simulink model "LoadFlow116BusNetwork_original"  (R2024a)
settings: Solver=FixedStepDiscrete  StartTime=0.0  StopTime=4.5  FixedStep=75e-6  RelTol=1e-3  EnableMultiTasking=on
undefined symbols (not defined in the file or in its folder): D1, D11, Delta
libraries: spsSeriesRLCBranchLib x164, spsLoadFlowBusLib x116, spsDistributedParametersLineLib x79, spsThreePhaseSeriesRLCLoadLib x60, spsThreePhaseTransformerTwoWindingsLib x52, spsThreePhaseParallelRLCLoadLib x44, spsThreePhaseVIMeasurementLib x44, spsSynchronousMachinepuStandardLib x28, spsExcitationSystemLib x28, spsHydraulicTurbineandGovernorLib x28, spsGenericPowerSystemStabilizerLib x28, spsMultiBandPowerSystemStabilizerLib x28
(part 7 of 15)

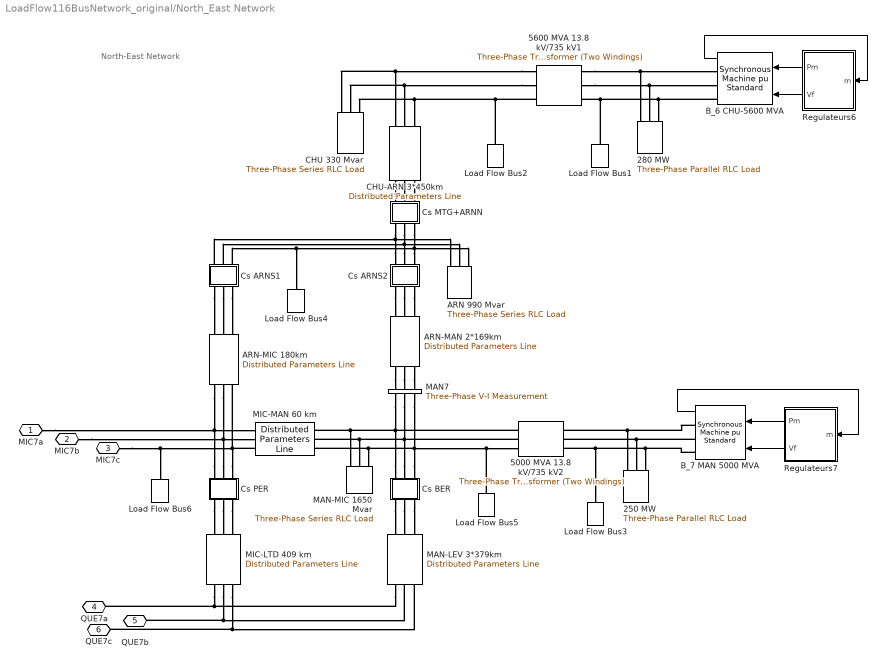
== system LoadFlow116BusNetwork_original/North_East Network ==
  note: North-East Network
  250 MW : spsThreePhaseParallelRLCLoadLib/Three-Phase Parallel RLC Load  LConnTagsString=A|B|C  Configuration=Y (grounded)  NominalVoltage=(13800)*1  Vabc=[1e3 1e3 1e3]  Vabcp=[1e3 1e3 1e3]  NominalFrequency=60  UnbalancedPower=off  ActivePower=250000000  InductivePower=0  CapacitivePower=0  Pabc=[10e3 9e3 11e3]  QLabc=[100 90 110]  QCabc=[100 90 110]  Pabcp=[10e3 9e3 11e3]  QLabcp=[100 90 110]  QCabcp=[100 90 110]  Measurements=None  LoadType=constant PQ
  280 MW : spsThreePhaseParallelRLCLoadLib/Three-Phase Parallel RLC Load  LConnTagsString=A|B|C  Configuration=Y (grounded)  NominalVoltage=(13800)*1  Vabc=[1e3 1e3 1e3]  Vabcp=[1e3 1e3 1e3]  NominalFrequency=60  UnbalancedPower=off  ActivePower=280000000  InductivePower=0  CapacitivePower=0  Pabc=[10e3 9e3 11e3]  QLabc=[100 90 110]  QCabc=[100 90 110]  Pabcp=[10e3 9e3 11e3]  QLabcp=[100 90 110]  QCabcp=[100 90 110]  Measurements=None  LoadType=constant PQ
  5000 MVA 13.8 kV/735 kV2 : spsThreePhaseTransformerTwoWindingsLib/Three-Phase Transformer (Two Windings)  Winding1Connection=Delta (D1)  Winding2Connection=Yg  CoreType=Three single-phase transformers  SetSaturation=off  Hysteresis=off  DataFile='basic_model'  SetInitialFlux=off  Measurements=None  UNITS=pu  NominalPower=[ 5000e6 60 ]  Winding1="[ 13.8e3 0.002  0.0]"  Winding2=[ 735e3 0.002 0.12]  Rm=500  Lm=500  L0=0.5  Saturation="[ 0,0  ;  0.005,1.2  ;  1.0,1.4 ]"  InitialFluxes=[ 0.8 , -0.8 , 0.7 ]  BreakLoop=off  DiscreteSolver=Trapezoidal iterative  DataType=off  TransfoNumber=0
  5600 MVA 13.8 kV/735 kV1 : spsThreePhaseTransformerTwoWindingsLib/Three-Phase Transformer (Two Windings)  Winding1Connection=Delta (D1)  Winding2Connection=Yg  CoreType=Three single-phase transformers  SetSaturation=off  Hysteresis=off  DataFile='basic_model'  SetInitialFlux=off  Measurements=None  UNITS=pu  NominalPower=[ 5600e6 60 ]  Winding1="[ 13.8e3 0.002  0.0]"  Winding2=[ 735e3 0.002 0.12]  Rm=500  Lm=500  L0=0.5  Saturation="[ 0,0  ;  0.005,1.2  ;  1.0,1.4 ]"  InitialFluxes=[ 0.8 , -0.8 , 0.7 ]  BreakLoop=off  DiscreteSolver=Trapezoidal iterative  DataType=off  TransfoNumber=0
  ARN 990 Mvar : spsThreePhaseSeriesRLCLoadLib/Three-Phase Series RLC Load  LConnTagsString=A|B|C  Configuration=Y (grounded)  NominalVoltage=735e3  Vabc=[1e3 1e3 1e3]  Vabcp=[1e3 1e3 1e3]  NominalFrequency=60  UnbalancedPower=off  ActivePower=3300000  InductivePower=990e6  CapacitivePower=0  Pabc=[10e3 9e3 11e3]  QLabc=[100 90 110]  QCabc=[100 90 110]  Pabcp=[10e3 9e3 11e3]  QLabcp=[100 90 110]  QCabcp=[100 90 110]  Measurements=None  LoadType=constant Z
  ARN-MAN 2*169km : spsDistributedParametersLineLib/Distributed Parameters Line  Phases=3  Length=169  Frequency=60  Resistance="[0.01273  0.3864]/2"  Inductance="[0.9337e-3  4.1264e-3]/2"  Capacitance=[12.74e-9 7.751e-9]*2  x1=[-0.000975 2.14769495598361e-09 336881.671287539 -573361.279314255;-0.0009 2.02121360131088e-09 352956.287913101 -563608.347624819;-0.000825 1.89311651941086e-09 368748.756682517 -553404.876045788;-0.00075 1.76350610913089e-09 384246.453337887 -542759.021076225;-0.000675 1.63248597904982e-09 399436.989257627 -531679.292849705;-0.0006 1.50016086465497e-09 414308.221359744 -520174.548331447;-0.000525 1.36663654461815e-09 428848.261808835 -508253.98423819;-0.00045 1.2320197562378e-09 443045.487519035 -495927.12968648;-0.000375 1.09641811011485e-09 456888.549445335 -483203.838575238;-0.0003 9.59940004130433e-10 470366.381655838 -470094.281708706;-0.000225 8.22694536794289e-10 483468.210177692 -456608.938666059;-0.00015 6.84791420033079e-10 496183.561609642 -442758.589424194;-7.5e-05 5.46340891488355e-10 508502.271494303 -428554.305740377]  x2=[-0.000975 1.31011450752005e-09 221203.742400063 -593985.664844247;-0.0009 1.1607432217342e-09 237907.645286858 -587494.731105769;-0.000825 1.01044405557687e-09 254421.36844212 -580534.163068216;-0.00075 8.59337155901819e-10 270731.711048227 -573109.524903176;-0.000675 7.0754331525264e-10 286825.634866856 -565226.751752799;-0.0006 5.55183875303024e-10 302690.274661552 -556892.14498533;-0.000525 4.02380629858089e-10 318312.948482 -548112.367157895;-0.00045 2.49255727494275e-10 333681.167801783 -538894.436690554;-0.000375 9.59315739156434e-11 348782.647501518 -529245.722255885;-0.0003 -5.74692658953743e-11 363605.315689394 -519173.936888575;-0.000225 -2.10824165654544e-10 378137.323351256 -508687.131819744;-0.00015 -3.64010535801408e-10 392367.053822526 -497793.690040911;-7.5e-05 -5.16905921495501e-10 406283.132074387 -486502.319602757]  x3=[-0.000975 1.18283624881266e-11 1173.57899596837 -608.931387386718;-0.0009 1.12673941317411e-11 1190.32360835483 -575.5111453786;-0.000825 1.06974187928836e-11 1206.11669426134 -541.630848566482;-0.00075 1.01188921011191e-11 1220.94562893665 -507.317580341249;-0.000675 9.53227652183314e-12 1234.79855835729 -472.598770204511;-0.0006 8.93804098654439e-12 1247.66440870343 -437.502171841875;-0.000525 8.33666051804761e-12 1259.53289521116 -402.055840937077;-0.00045 7.72861585068788e-12 1270.39453039396 -366.288112744694;-0.000375 7.1143930460689e-12 1280.24063162684 -330.227579439379;-0.0003 6.49448310450276e-12 1289.06332808715 -293.903067259712;-0.000225 5.8693815725118e-12 1296.85556704631 -257.343613464944;-0.00015 5.23958814669633e-12 1303.61111950773 -220.578443123063;-7.5e-05 4.60560627428477e-12 1309.32458518613 -183.636945748712]  x4=[-0.000975 -2.47161415316379e-13 1977.2372844662 -8416.68856749833;-0.0009 -4.34177553917464e-13 2214.39295528633 -8357.42673046412;-0.000825 -6.20846617625088e-13 2449.77847425936 -8291.48409437449;-0.00075 -8.07019386045854e-13 2683.20567780293 -8218.91337276378;-0.000675 -9.92547035517226e-13 2914.48796778209 -8139.77257755647;-0.0006 -1.17728125807488e-12 3143.44046067297 -8054.12497269336;-0.000525 -1.36107438000785e-12 3369.88013535583 -7962.03902355932;-0.00045 -1.54377947990656e-12 3593.62597941939 -7863.58834225313;-0.000375 -1.72525050610966e-12 3814.49913385932 -7758.85162874308;-0.0003 -1.9053423934554e-12 4032.32303605544 -7647.91260795543;-0.000225 -2.08391117924452e-12 4246.92356091315 -7530.85996284596;-0.00015 -2.26081411832186e-12 4458.12916005637 -7407.78726350822;-7.5e-05 -2.43590979718463e-12 4665.77099896071 -7278.79289237497]  x5=0.000955765248222805  V1=ones(3,3)  V2=ones(3,3)  I1=ones(3,3)  I2=ones(3,3)  nHarmo=1  Measurements=None  Decoupling=off  VsMag0=[ 1 1 1]  VrMag0=[ 1 1 1]  VsAngle0=[0 -120 120]  VrAngle0=[0 -120 120]  IsMag0=[ 1 1 1]  IrMag0=[ 1 1 1]  IsAngle0=[0 -120 120]  IrAngle0=[0 -120 120]
      settings: AttributesFormatString=\n  LibrarySourceBlock=sps_lib/Power Grid Elements/Distributed Parameters Line
  ARN-MIC 180km : spsDistributedParametersLineLib/Distributed Parameters Line  Phases=3  Length=180  Frequency=60  Resistance="[0.01273  0.3864]"  Inductance="[0.9337e-3  4.1264e-3]"  Capacitance=[12.74e-9 7.751e-9]  x1=[-0.00105 2.02356997613359e-09 327893.271560195 -568370.375306617;-0.000975 1.90934055554331e-09 343830.386178329 -558873.543001994;-0.0009 1.79358483732682e-09 359492.648046534 -548929.955738147;-0.000825 1.67639535483414e-09 374867.536992312 -538547.562266593;-0.00075 1.55786578754451e-09 389942.762564684 -527734.662113816;-0.000675 1.43809088618047e-09 404706.273858986 -516499.898946758;-0.0006 1.31716639696554e-09 419146.269150178 -504852.253663194;-0.000525 1.19518898508619e-09 433251.205326966 -492801.037212551;-0.00045 1.07225615741918e-09 447009.80711918 -480355.883152868;-0.000375 9.48466184585991e-10 460411.076111063 -467526.739949885;-0.0003 8.23918022396866e-10 473444.299533228 -454323.863024385;-0.000225 6.98711232747004e-10 486099.058826288 -440757.806554171;-0.00015 5.72945904028325e-10 498365.237969286 -426839.415037219;-7.5e-05 4.46722571120333e-10 510233.031566296 -412579.814622748]  x2=[-0.00105 6.51645326703719e-09 183777.347501457 -621430.39717543;-0.000975 6.348283068608e-09 201272.089254488 -615986.55973462;-0.0009 6.17503814982576e-09 218605.937178935 -610050.312062869;-0.000825 5.9968570000278e-09 235765.034861984 -603626.399505737;-0.00075 5.813882054499e-09 252735.665583491 -596719.957240634;-0.000675 5.62625958061122e-09 269504.263280915 -589336.506171834;-0.0006 5.43413956089935e-09 286057.423393827 -581481.948517152;-0.000525 5.23767557316763e-09 302381.913579302 -573162.563089797;-0.00045 5.03702466772183e-09 318464.684289661 -564385.000279189;-0.000375 4.83234724182573e-09 334292.879204071 -555156.276734738;-0.0003 4.6238069114819e-09 349853.845505699 -545483.769756842;-0.000225 4.41157038063965e-09 365135.143996172 -535375.211399583;-0.00015 4.1958073079344e-09 380124.55903929 -524838.682289847;-7.5e-05 3.9766901710652e-09 394810.108326013 -513882.60516779]  x3=[-0.00105 1.31803756803945e-11 35.6370942885461 24.8424671156337;-0.000975 1.34306150989482e-11 34.9200556852133 25.8396049019067;-0.0009 1.3670118289287e-11 34.1751025236605 26.8160869033804;-0.000825 1.38986937962253e-11 33.4028303080469 27.7711325352834;-0.00075 1.41161589e-11 32.6038563809654 28.7039783487503;-0.000675 1.43223397623345e-11 31.7788194299488 29.6138786411108;-0.0006 1.45170715654021e-11 30.9283789769121 30.5001060519931;-0.000525 1.4700198643579e-11 30.0532148509414 31.3619521447648;-0.00045 1.48715746078808e-11 29.1540266448484 32.1987279728458;-0.000375 1.50310624629838e-11 28.231533155927 33.0097646304425;-0.0003 1.51785347167368e-11 27.2864718113578 33.7944137872598;-0.000225 1.53138734820767e-11 26.3195980787196 34.5520482067676;-0.00015 1.54369705712651e-11 25.3316848620806 35.2820622476029;-7.5e-05 1.55477275823724e-11 24.3235218841506 35.9838723477111]  x4=[-0.00105 1.50447165715535e-12 1327.91429807042 -4613.12548250188;-0.000975 9.57042222094167e-13 1457.79983330366 -4573.74071492918;-0.0009 4.08847742123886e-13 1586.52002565523 -4530.69976900954;-0.000825 -1.3967356447587e-13 1713.97197817287 -4484.03705101658;-0.00075 -6.88083218165262e-13 1840.0538077158 -4433.78986241311;-0.000675 -1.23594282865808e-12 1964.66472639862 -4379.99837003289;-0.0006 -1.78281444536423e-12 2087.70512215952 -4322.70557397188;-0.000525 -2.32826090748072e-12 2209.07663838874 -4261.95727321466;-0.00045 -2.87184619345137e-12 2328.68225255323 -4197.80202902336;-0.000375 -3.41313576951569e-12 2446.42635375507 -4130.29112611858;-0.0003 -3.95169693706859e-12 2562.21481916129 -4059.47853168316;-0.000225 -4.48709917855298e-12 2675.95508924428 -3985.42085222162;-0.00015 -5.01891450160896e-12 2787.5562417724 -3908.17728830979;-7.5e-05 -5.54671778120432e-12 2896.9290644919 -3827.8095872708]  x5=0.00101797482059234  V1=ones(3,3)  V2=ones(3,3)  I1=ones(3,3)  I2=ones(3,3)  nHarmo=1  Measurements=None  Decoupling=off  VsMag0=[ 1 1 1]  VrMag0=[ 1 1 1]  VsAngle0=[0 -120 120]  VrAngle0=[0 -120 120]  IsMag0=[ 1 1 1]  IrMag0=[ 1 1 1]  IsAngle0=[0 -120 120]  IrAngle0=[0 -120 120]
      settings: AttributesFormatString=\n  LibrarySourceBlock=sps_lib/Power Grid Elements/Distributed Parameters Line
  "B_6 CHU-5600 MVA " : spsSynchronousMachinepuStandardLib/Synchronous Machine pu Standard  PresetModel=No  MechanicalLoad=Mechanical power Pm  ShowDetailedParameters=on  RotorType=Salient-pole  Units=per unit standard parameters  MeasurementBus=off  NominalParameters="[ 5600E6  13800   60 ]"  Reactances1=[ 31 32 33 34 35 36 37 ]  Reactances2=[ 1.305, 0.296, 0.252, 0.474, 0.243, 0.18 ]  dAxisTimeConstants=Short-circuit  qAxisTimeConstants=Open-circuit  TimeConstants1=[]  TimeConstants2=[]  TimeConstants3=[]  TimeConstants4=[]  TimeConstants5=[ 1.01, 0.053, 0.1 ]  TimeConstants6=[]  TimeConstants7=[]  TimeConstants8=[]  StatorResistance=2.8544e-3  Mechanical="[ 4.0 0  32]"  PolePairs=32  InitialConditions=[0 -61.7964 0.894782 0.894782 0.894782 8.48442 -111.516 128.484 1.31361]  SetSaturation=off  Saturation=[0.6404,0.7127,0.8441,0.9214,0.9956,1.082,1.19,1.316,1.457;0.7,0.7698,0.8872,0.9466,0.9969,1.046,1.1,1.151,1.201]  LoadFlowParameters=[1 5000000000 0 0 0]  TsPowergui=0  TsBlock=-1  IterativeModel=Trapezoidal non iterative  IterativeDiscreteModel=Trapezoidal non iterative  BusType=PV  Pref=5000000000  Qref=0  Qmin=-Inf  Qmax=Inf  PLF=0  QLF=0
  B_7 MAN 5000 MVA : spsSynchronousMachinepuStandardLib/Synchronous Machine pu Standard  PresetModel=No  MechanicalLoad=Mechanical power Pm  ShowDetailedParameters=on  RotorType=Salient-pole  Units=per unit standard parameters  MeasurementBus=off  NominalParameters="[ 5000E6  13800   60 ]"  Reactances1=[ 31 32 33 34 35 36 37 ]  Reactances2=[ 1.305, 0.296, 0.252, 0.474, 0.243, 0.18 ]  dAxisTimeConstants=Short-circuit  qAxisTimeConstants=Open-circuit  TimeConstants1=[]  TimeConstants2=[]  TimeConstants3=[]  TimeConstants4=[]  TimeConstants5=[ 1.01, 0.053, 0.1 ]  TimeConstants6=[]  TimeConstants7=[]  TimeConstants8=[]  StatorResistance=2.8544e-3  Mechanical="[ 3.7 0  32]"  PolePairs=32  InitialConditions=[0 -81.9543 0.907703 0.907703 0.907703 -8.76021 -128.76 111.24 1.25655]  SetSaturation=off  Saturation=[0.6404,0.7127,0.8441,0.9214,0.9956,1.082,1.19,1.316,1.457;0.7,0.7698,0.8872,0.9466,0.9969,1.046,1.1,1.151,1.201]  LoadFlowParameters=[1 4500000000 0 0 0]  TsPowergui=0  TsBlock=-1  IterativeModel=Trapezoidal non iterative  IterativeDiscreteModel=Trapezoidal non iterative  BusType=PV  Pref=4500000000  Qref=0  Qmin=-Inf  Qmax=Inf  PLF=0  QLF=0
  CHU 330 Mvar : spsThreePhaseSeriesRLCLoadLib/Three-Phase Series RLC Load  LConnTagsString=A|B|C  Configuration=Y (grounded)  NominalVoltage=735e3  Vabc=[1e3 1e3 1e3]  Vabcp=[1e3 1e3 1e3]  NominalFrequency=60  UnbalancedPower=off  ActivePower=1100000  InductivePower=330e6  CapacitivePower=0  Pabc=[10e3 9e3 11e3]  QLabc=[100 90 110]  QCabc=[100 90 110]  Pabcp=[10e3 9e3 11e3]  QLabcp=[100 90 110]  QCabcp=[100 90 110]  Measurements=None  LoadType=constant Z
  CHU-ARN 3*450km : spsDistributedParametersLineLib/Distributed Parameters Line  Phases=3  Length=450  Frequency=60  Resistance="[0.01273  0.3864]/3"  Inductance="[0.9337e-3  4.1264e-3]/3"  Capacitance=[12.74e-9 7.751e-9]*3  x1=[-0.00255 1.20759491790477e-09 0 0;-0.002475 1.18127165846567e-09 0 0;-0.0024 1.15400410853686e-09 0 0;-0.002325 1.12581406538053e-09 0 0;-0.00225 1.09672406368588e-09 0 0;-0.002175 1.06675735755515e-09 0 0;-0.0021 1.03593790191473e-09 0 0;-0.002025 1.00429033336591e-09 0 0;-0.00195 9.71839950490742e-10 0 0;-0.001875 9.38612693628805e-10 0 0;-0.0018 9.04635124140838e-10 0 0;-0.001725 8.69934403176013e-10 0 0;-0.00165 8.34538269959732e-10 0 0;-0.001575 7.9847501961931e-10 351966.370721147 -543333.024589086;-0.0015 7.61773480565281e-10 367186.081536688 -533165.672905933;-0.001425 7.24462991446413e-10 382112.269416784 -522572.116741568;-0.00135 6.86573377696839e-10 396733.002595223 -511560.8244227;-0.001275 6.48134927694059e-10 411036.593481605 -500140.598207933;-0.0012 6.09178368546877e-10 425011.608004229 -488320.567251365;-0.001125 5.6973484153262e-10 438646.874750309 -476110.180304892;-0.00105 5.29835877203277e-10 451931.493896237 -463519.198165013;-0.000975 4.89513370180459e-10 464854.845920728 -450557.685870203;-0.0009 4.48799553659325e-10 477406.600093907 -437236.004655072;-0.000825 4.07726973641858e-10 489576.722735537 -423564.803667755;-0.00075 3.66328462920094e-10 501355.485235788 -409555.011457145;-0.000675 3.24637114830086e-10 512733.471832137 -395217.827236777;-0.0006 2.82686256797596e-10 523701.587136189 -380564.711932352;-0.000525 2.40509423696668e-10 534251.063404387 -365607.379020044;-0.00045 1.98140331042353e-10 544373.467546815 -350357.785162928;-0.000375 1.55612848039052e-10 554060.707868479 -334828.120653006;-0.0003 1.12960970505986e-10 563305.040537687 -319030.799666476;-0.000225 7.02187937014572e-11 572099.075776344 -302978.450340028;-0.00015 2.74204850676273e-11 580435.783767236 -286683.904676103;-7.5e-05 -1.53997430824181e-11 588308.500273549 -270160.188285192]  x2=[-0.00255 3.7772292779939e-09 0 0;-0.002475 3.71020134114714e-09 0 0;-0.0024 3.64020752611626e-09 0 0;-0.002325 3.56730378488603e-09 0 0;-0.00225 3.49154839559175e-09 0 0;-0.002175 3.41300191593251e-09 0 0;-0.0021 3.33172713476236e-09 0 0;-0.002025 3.24778902189781e-09 0 0;-0.00195 3.161254676182e-09 0 0;-0.001875 3.07219327184686e-09 0 0;-0.0018 2.98067600321635e-09 0 0;-0.001725 2.88677602779473e-09 0 0;-0.00165 2.79056840778565e-09 0 0;-0.001575 2.69213005008852e-09 34511.8097316948 -640486.415414501;-0.0015 2.59153964482031e-09 52604.9373493269 -639254.768695303;-0.001425 2.48887760241192e-09 70656.0133849246 -637512.111494935;-0.00135 2.38422598932927e-09 88650.6080844956 -635259.836866901;-0.001275 2.27766846247063e-09 106574.336844364 -632499.745245077;-0.0012 2.16929020229259e-09 124412.87171 -629234.043004475;-0.001125 2.05917784471808e-09 142151.952829573 -625465.340697498;-0.00105 1.94741941188099e-09 159777.399853051 -621196.650967109;-0.000975 1.83410424176256e-09 177275.123267763 -616431.386138564;-0.0009 1.71932291677599e-09 194631.135661335 -611173.355491656;-0.000825 1.60316719135628e-09 211831.562903016 -605426.762215634;-0.00075 1.48572991861308e-09 228862.655234444 -599196.200049237;-0.000675 1.36710497610537e-09 245710.798260993 -592486.64960853;-0.0006 1.24738719079717e-09 262362.523834914 -585303.474405476;-0.000525 1.12667226325431e-09 278804.520821562 -577652.416560425;-0.00045 1.00505669114286e-09 295023.645740118 -569539.592211955;-0.000375 8.82637692090403e-10 311006.933270282 -560971.486627718;-0.0003 7.59513125971696e-10 326741.606616555 -551954.949020222;-0.000225 6.35781416681028e-10 342215.087721814 -542497.187071674;-0.00015 5.11541473453646e-10 357415.007322014 -532605.761172266;-7.5e-05 3.86892611799233e-10 372329.214833994 -522288.578376518]  x3=[-0.00255 1.3083615183075e-11 0 0;-0.002475 1.33054726191203e-11 0 0;-0.0024 1.35166938639345e-11 0 0;-0.002325 1.37171100704862e-11 0 0;-0.00225 1.39065610291264e-11 0 0;-0.002175 1.40848952956574e-11 0 0;-0.0021 1.42519703123952e-11 0 0;-0.002025 1.44076525221277e-11 0 0;-0.00195 1.45518174748785e-11 0 0;-0.001875 1.46843499273902e-11 0 0;-0.0018 1.4805143935248e-11 0 0;-0.001725 1.49141029375702e-11 0 0;-0.00165 1.50111398341976e-11 0 0;-0.001575 1.50961770553197e-11 -94.847357634225 -855.378108344289;-0.0015 1.5169146623483e-11 -70.6281637613808 -857.719458193193;-0.001425 1.52299902079312e-11 -46.3525108150729 -859.375160230765;-0.00135 1.52786591712339e-11 -22.0398043808365 -860.34389091413;-0.001275 1.53151146081664e-11 2.29052033580138 -860.624875854801;-0.0012 1.53393273768102e-11 26.6190140455292 -860.217890437716;-0.001125 1.53512781218486e-11 50.9262289227134 -859.12326000079;-0.00105 1.53509572900389e-11 75.1927341516944 -857.341859574846;-0.000975 1.53383651378489e-11 99.3991314594819 -854.875113184128;-0.0009 1.53135117312527e-11 123.526070622438 -851.724992707958;-0.000825 1.52764169376831e-11 147.554264934551 -847.894016304448;-0.00075 1.52271104101505e-11 171.464506624932 -843.385246397517;-0.000675 1.51656315635386e-11 195.237682212211 -838.202287228842;-0.0006 1.50920295430968e-11 218.854787783567 -832.349281976682;-0.000525 1.5006363185154e-11 242.296944186159 -825.830909443881;-0.00045 1.49087009700861e-11 265.545412118836 -818.652380317708;-0.000375 1.47991209675735e-11 288.581607112046 -810.819433004509;-0.0003 1.46777107741935e-11 311.387114383978 -802.33832904252;-0.000225 1.45445674433972e-11 333.943703561054 -793.215848096483;-0.00015 1.43997974079259e-11 356.233343251013 -783.459282538087;-7.5e-05 1.4243516394731e-11 378.23821545693 -773.076431616559]  x4=[-0.00255 9.80324671229956e-12 0 0;-0.002475 9.4388577764635e-12 0 0;-0.0024 9.06692356214031e-12 0 0;-0.002325 8.68774138785012e-12 0 0;-0.00225 8.30161436602138e-12 0 0;-0.002175 7.90885116068741e-12 0 0;-0.0021 7.50976574074506e-12 0 0;-0.002025 7.10467712897283e-12 0 0;-0.00195 6.6939091470089e-12 0 0;-0.001875 6.27779015649311e-12 0 0;-0.0018 5.85665279657962e-12 0 0;-0.001725 5.43083371803033e-12 0 0;-0.00165 5.0006733141014e-12 0 0;-0.001575 4.56651544843804e-12 398.583364810219 -13326.9833161375;-0.0015 4.12870718019523e-12 775.187270558394 -13310.3877177117;-0.001425 3.68759848660391e-12 1151.17150346325 -13283.1519990002;-0.00135 3.24354198320454e-12 1526.23550748175 -13245.2979318198;-0.001275 2.79689264197166e-12 1900.07946218775 -13196.8557761325;-0.0012 2.34800750755468e-12 2272.40452244388 -13137.8642558564;-0.001125 1.89724541186188e-12 2642.91305729371 -13068.3705279103;-0.00105 1.44496668721567e-12 3011.30888788347 -12988.4301445169;-0.000975 9.91532878308424e-13 3377.29752422283 -12898.1070087956;-0.0009 5.37306453189224e-13 3740.58640059571 -12797.4733236792;-0.000825 8.26505135124086e-14 4100.88510943285 -12686.6095341957;-0.00075 -3.72071495720313e-13 4457.90563345915 -12565.6042631622;-0.000675 -8.26496076692243e-13 4811.3625759303 -12434.554240341;-0.0006 -1.28025996934628e-12 5160.97338877458 -12293.564225115;-0.000525 -1.73300044176945e-12 5506.4585984574 -12142.7469227454;-0.00045 -2.18435558015527e-12 5847.54202938827 -11982.2228942759;-0.000375 -2.63396457811207e-12 6183.95102469123 -11812.120460159;-0.0003 -3.08146802508614e-12 6515.41666416268 -11632.5755976777;-0.000225 -3.526508193669e-12 6841.67397924201 -11443.731832248;-0.00015 -3.96872932555923e-12 7162.46216482347 -11245.7401226865;-7.5e-05 -4.40777791595019e-12 7477.5247877397 -11038.7587405366]  x5=0.00254493705148084  V1=ones(3,3)  V2=ones(3,3)  I1=ones(3,3)  I2=ones(3,3)  nHarmo=1  Measurements=None  Decoupling=off  VsMag0=[ 1 1 1]  VrMag0=[ 1 1 1]  VsAngle0=[0 -120 120]  VrAngle0=[0 -120 120]  IsMag0=[ 1 1 1]  IrMag0=[ 1 1 1]  IsAngle0=[0 -120 120]  IrAngle0=[0 -120 120]
      settings: AttributesFormatString=\n  LibrarySourceBlock=sps_lib/Power Grid Elements/Distributed Parameters Line
  "Cs ARNS1 " : Subsystem  mask{Xc=25}
      mask prompts: Xc "Condensator Reactance at  60Hz  (ohm):"
      mask help: Series Compensation
      mask init:
      | Cs=1/Xc/(2*pi*60);
      mask Display: disp('Cs')
  Cs ARNS2 : Subsystem  mask{Xc=25/2}
      mask prompts: Xc "Condensator Reactance at  60Hz  (ohm):"
      mask help: Series Compensation
      mask init:
      | Cs=1/Xc/(2*pi*60);
      mask Display: disp('Cs')
  Cs BER : Subsystem  mask{Xc=22/3}
      mask prompts: Xc "Condensator Reactance at  60Hz  (ohm):"
      mask help: Series Compensation
      mask init:
      | Cs=1/Xc/(2*pi*60);
      mask Display: disp('Cs')
  "Cs MTG+ARNN " : Subsystem  mask{Xc=(30+25)/3}
      mask prompts: Xc "Condensator Reactance at  60Hz  (ohm):"
      mask help: Series Compensation
      mask init:
      | Cs=1/Xc/(2*pi*60);
      mask Display: disp('Cs')
  "Cs PER " : Subsystem  mask{Xc=22}
      mask prompts: Xc "Condensator Reactance at  60Hz  (ohm):"
      mask help: Series Compensation
      mask init:
      | Cs=1/Xc/(2*pi*60);
      mask Display: disp('Cs')
  Load Flow Bus1 : spsLoadFlowBusLib/Load Flow Bus  LConnTagsString=a  Phases=single  Connectors=on one side  ID=CHU_13.8  Vbase=13.8e3  Vref=1  Vangle=0  VLF=1  VLFb=1  VLFc=1  angleLF=4.726  angleLFb=0  angleLFc=0
      settings: AttributesFormatString=%<ID>\n%<Vbase>V\n%<VLF>pu\n%<angleLF>deg.
  Load Flow Bus2 : spsLoadFlowBusLib/Load Flow Bus  LConnTagsString=a  Phases=single  Connectors=on one side  ID=CHU7  Vbase=735e3  Vref=1  Vangle=0  VLF=1.009  VLFb=1  VLFc=1  angleLF=28.97  angleLFb=0  angleLFc=0
      settings: AttributesFormatString=%<ID>\n%<Vbase>V\n%<VLF>pu\n%<angleLF>deg.
  Load Flow Bus3 : spsLoadFlowBusLib/Load Flow Bus  LConnTagsString=a  Phases=single  Connectors=on one side  ID=MAN_13.8  Vbase=13.8e3  Vref=1  Vangle=0  VLF=1  VLFb=1  VLFc=1  angleLF=-16.23  angleLFb=0  angleLFc=0
      settings: AttributesFormatString=%<ID>\n%<Vbase>V\n%<VLF>pu\n%<angleLF>deg.
  Load Flow Bus4 : spsLoadFlowBusLib/Load Flow Bus  LConnTagsString=a  Phases=single  Connectors=on one side  ID=ARN7  Vbase=735e3  Vref=1  Vangle=0  VLF=1.054  VLFb=1  VLFc=1  angleLF=12.72  angleLFb=0  angleLFc=0
      settings: AttributesFormatString=%<ID>\n%<Vbase>V\n%<VLF>pu\n%<angleLF>deg.
  Load Flow Bus5 : spsLoadFlowBusLib/Load Flow Bus  LConnTagsString=a  Phases=single  Connectors=on one side  ID=MAN7  Vbase=735e3  Vref=1  Vangle=0  VLF=1.016  VLFb=1  VLFc=1  angleLF=7.996  angleLFb=0  angleLFc=0
      settings: AttributesFormatString=%<ID>\n%<Vbase>V\n%<VLF>pu\n%<angleLF>deg.
  Load Flow Bus6 : spsLoadFlowBusLib/Load Flow Bus  LConnTagsString=a  Phases=single  Connectors=on one side  ID=MIC7  Vbase=735e3  Vref=1  Vangle=0  VLF=1.041  VLFb=1  VLFc=1  angleLF=5.981  angleLFb=0  angleLFc=0
      settings: AttributesFormatString=%<ID>\n%<Vbase>V\n%<VLF>pu\n%<angleLF>deg.
  MAN-LEV 3*379km : spsDistributedParametersLineLib/Distributed Parameters Line  Phases=3  Length=379  Frequency=60  Resistance="[0.01273  0.3864]/3"  Inductance="[0.9337e-3  4.1264e-3]/3"  Capacitance=[12.74e-9 7.751e-9]*3  x1=[-0.002175 3.68092852673604e-09 2062.13690456457 -628964.364618891;-0.0021 3.64987273995699e-09 19842.5129724228 -628654.706299026;-0.002025 3.61589930075454e-09 37607.0272390116 -627842.511025686;-0.00195 3.57903536697618e-09 55341.4790234324 -626528.428055344;-0.001875 3.53931040708655e-09 73031.6916762748 -624713.507845821;-0.0018 3.49675617661075e-09 90663.5239122135 -622399.201216563;-0.001725 3.45140669274953e-09 108222.881114335 -619587.358188879;-0.00165 3.40329820718643e-09 125695.72660116 -616280.226507064;-0.001575 3.3524691771087e-09 143068.092847349 -612480.449841583;-0.0015 3.2989602344653e-09 160326.09264913 -608191.065675764;-0.001425 3.24281415348624e-09 177455.93022552 -603415.502877679;-0.00135 3.18407581648961e-09 194443.912246454 -598157.57895916;-0.001275 3.12279217800328e-09 211276.45877903 -592421.497024139;-0.0012 3.05901222723016e-09 227940.114143096 -586211.84240875;-0.001125 2.99278694888706e-09 244421.557667517 -579533.579015881;-0.00105 2.92416928244819e-09 260707.614338513 -572392.045347108;-0.000975 2.85321407982623e-09 276785.265331568 -564792.950235177;-0.0009 2.77997806152449e-09 292641.658418473 -556742.368280449;-0.000825 2.70451977129546e-09 308264.118241206 -548246.734994962;-0.00075 2.62689952934179e-09 323640.156444416 -539312.841657977;-0.000675 2.54717938409728e-09 338757.481658425 -529947.829887133;-0.0006 2.46542306262628e-09 353604.00932476 -520159.185929551;-0.000525 2.38169591968125e-09 368167.871356363 -509954.73467744;-0.00045 2.29606488545919e-09 382437.425624761 -499342.633412996;-0.000375 2.20859841209867e-09 396401.265266603 -488331.365287601;-0.0003 2.11936641896021e-09 410048.227802135 -476929.732540515;-0.000225 2.02844023673382e-09 423367.404058309 -465146.849462505;-0.00015 1.93589255041837e-09 436348.146889418 -452992.135110021;-7.5e-05 1.84179734121826e-09 448980.079688253 -440475.305775742]  x2=[-0.002175 2.01856949538252e-08 -361248.126814235 -552999.635419905;-0.0021 2.0189787521832e-08 -345470.121722022 -562991.298925658;-0.002025 2.0177740682608e-08 -329415.953100374 -572532.915801107;-0.00195 2.0149564066212e-08 -313098.45440605 -581616.858623711;-0.001875 2.01052801966003e-08 -296530.669597842 -590235.865828568;-0.0018 2.00449244736204e-08 -279725.842709428 -598383.047513193;-0.001725 1.9968545144714e-08 -262697.407262301 -606051.890945204;-0.00165 1.98762032663479e-08 -245458.975527214 -613236.265768497;-0.001575 1.97679726552067e-08 -228024.327642739 -619930.428903766;-0.0015 1.96439398291852e-08 -210407.400599635 -626129.029139422;-0.001425 1.95042039382265e-08 -192622.277099833 -631827.111409279;-0.00135 1.93488766850639e-08 -174683.174298938 -637020.120753555;-0.001275 1.91780822359271e-08 -156604.43244125 -641703.905960035;-0.0012 1.89919571212853e-08 -138400.503396396 -645874.72288249;-0.001125 1.87906501267075e-08 -120085.939106726 -649529.237433687;-0.00105 1.85743221739249e-08 -101675.379954711 -652664.52825061;-0.000975 1.83431461921932e-08 -83183.5430596452 -655278.089029752;-0.0009 1.8097306980055e-08 -64625.2105130086 -657367.830530614;-0.000825 1.7837001057615e-08 -46015.2175618868 -658932.082245816;-0.00075 1.75624365094449e-08 -27368.4407499025 -659969.593736469;-0.000675 1.72738328182434e-08 -8699.7860251338 -660479.535631762;-0.0006 1.69714206893854e-08 9975.82317547212 -660461.500291947;-0.000525 1.66554418664999e-08 28643.4578556668 -659915.502134199;-0.00045 1.6326148938223e-08 47288.1953939113 -658841.97762109;-0.000375 1.59838051362834e-08 65895.1314722915 -657241.784911691;-0.0003 1.56286841250783e-08 84449.3919908021 -655116.203175571;-0.000225 1.52610697829104e-08 102936.144957474 -652466.931570246;-0.00015 1.48812559750603e-08 121340.612344843 -649296.087882902;-7.5e-05 1.44895463188746e-08 139648.081903277 -645606.206837468]  x3=[-0.002175 2.56553598523634e-11 -242.422201517504 1603.55585538018;-0.0021 2.80158344409494e-11 -287.659078132665 1596.06084494524;-0.002025 3.035391360014e-11 -332.666004482099 1587.28996789141;-0.00195 3.26677283052291e-11 -377.40700271751 1577.2502355236;-0.001875 3.4955428928144e-11 -421.84630756947 1565.94967345024;-0.0018 3.72151867160097e-11 -465.948394937624 1553.39731516777;-0.001725 3.94451952530261e-11 -509.678010288114 1539.60319483932;-0.00165 4.1643671904489e-11 -553.000196835515 1524.57833927364;-0.001575 4.38088592418009e-11 -595.880323486752 1508.33475911037;-0.0015 4.5939026447333e-11 -638.284112524668 1490.88543921897;-0.001425 4.80324706980138e-11 -680.177667009107 1472.24432831876;-0.00135 5.008751852654e-11 -721.527497873606 1452.4263278286;-0.001275 5.21025271591208e-11 -762.300550696046 1431.44727995483;-0.0012 5.40758858286861e-11 -802.464232121849 1409.32395502735;-0.001125 5.60060170625086e-11 -841.986435918608 1386.0740380936;-0.00105 5.78913779432123e-11 -880.835568641318 1361.71611478143;-0.000975 5.97304613421558e-11 -918.980574887693 1336.26965644207;-0.0009 6.15217971242092e-11 -956.390962123377 1309.75500458496;-0.000825 6.32639533229566e-11 -993.036825057211 1282.19335461711;-0.00075 6.49555372853885e-11 -1028.88886954707 1253.60673889979;-0.000675 6.65951967851675e-11 -1063.91843601714 1224.01800913623;-0.0006 6.81816211035771e-11 -1098.09752236795 1193.45081810426;-0.000525 6.97135420772903e-11 -1131.39880636084 1161.92960074871;-0.00045 7.118973511212e-11 -1163.79566745891 1129.47955464844;-0.000375 7.26090201619404e-11 -1195.26220810708 1096.1266198738;-0.0003 7.39702626719986e-11 -1225.77327443421 1061.89745825054;-0.000225 7.52723744858599e-11 -1255.30447636072 1026.81943204672;-0.00015 7.65143147152631e-11 -1283.83220709563 990.920582099793;-7.5e-05 7.76950905721911e-11 -1311.33366200749 954.229605401126]  x4=[-0.002175 6.07610984127132e-11 -6948.98880273919 -13531.9699054556;-0.0021 5.93565147342189e-11 -6563.65417562416 -13723.0127844946;-0.002025 5.79044823660313e-11 -6173.07266378842 -13903.0856970828;-0.00195 5.64061620406085e-11 -5777.55649211642 -14072.0446956891;-0.001875 5.48627514922937e-11 -5377.42183018421 -14229.7547170752;-0.0018 5.32754844998642e-11 -4972.98853951826 -14376.089690263;-0.001725 5.16456299002677e-11 -4564.5799179031 -14510.932637314;-0.00165 4.99744905743336e-11 -4152.52244094197 -14634.1757668394;-0.001575 4.82634024052698e-11 -3737.14550107729 -14745.7205601672;-0.0015 4.6513733210778e-11 -3318.78114427928 -14845.4778500963;-0.001425 4.47268816496414e-11 -2897.7638046136 -14933.3678921755;-0.00135 4.29042761036584e-11 -2474.43003689977 -15009.3204284498;-0.001275 4.10473735358156e-11 -2049.1182476745 -15073.2747436239;-0.0012 3.91576583256141e-11 -1622.1684246746 -15125.1797135969;-0.001125 3.72366410824793e-11 -1193.92186505602 -15164.9938463297;-0.00105 3.5285857438203e-11 -764.720902566135 -15192.6853150141;-0.000975 3.33068668193823e-11 -334.908633887359 -15208.2319835134;-0.0009 3.13012512008383e-11 95.1713556290706 -15211.6214240589;-0.000825 2.92706138410096e-11 525.175266619982 -15202.8509271837;-0.00075 2.72165780003317e-11 954.759360538207 -15181.9275038886;-0.000675 2.5140785643628e-11 1383.58023443193 -15148.8678800382;-0.0006 2.30448961275478e-11 1811.29509545573 -15103.69848299;-0.000525 2.09305848741019e-11 2237.56203489397 -15046.4554204688;-0.00045 1.87995420313563e-11 2662.04030147736 -14977.184451703;-0.000375 1.66534711223535e-11 3084.39057377434 -14895.9409508451;-0.0003 1.44940876833421e-11 3504.27523143939 -14802.7898627066;-0.000225 1.23231178924037e-11 3921.35862510165 -14697.8056508422;-0.00015 1.0142297189572e-11 4335.30734467779 -14581.0722380244;-7.5e-05 7.95336888954945e-12 4745.79048589503 -14452.6829391574]  x5=0.00214340253891386  V1=ones(3,3)  V2=ones(3,3)  I1=ones(3,3)  I2=ones(3,3)  nHarmo=1  Measurements=None  Decoupling=off  VsMag0=[ 1 1 1]  VrMag0=[ 1 1 1]  VsAngle0=[0 -120 120]  VrAngle0=[0 -120 120]  IsMag0=[ 1 1 1]  IrMag0=[ 1 1 1]  IsAngle0=[0 -120 120]  IrAngle0=[0 -120 120]
      settings: AttributesFormatString=\n  LibrarySourceBlock=sps_lib/Power Grid Elements/Distributed Parameters Line
  MAN-MIC 1650 Mvar : spsThreePhaseSeriesRLCLoadLib/Three-Phase Series RLC Load  LConnTagsString=A|B|C  Configuration=Y (grounded)  NominalVoltage=735e3  Vabc=[1e3 1e3 1e3]  Vabcp=[1e3 1e3 1e3]  NominalFrequency=60  UnbalancedPower=off  ActivePower=5500000  InductivePower=1650e6  CapacitivePower=0  Pabc=[10e3 9e3 11e3]  QLabc=[100 90 110]  QCabc=[100 90 110]  Pabcp=[10e3 9e3 11e3]  QLabcp=[100 90 110]  QCabcp=[100 90 110]  Measurements=None  LoadType=constant Z
  MAN7 : spsThreePhaseVIMeasurementLib/Three-Phase V-I Measurement  VoltageMeasurement=no  SetLabelV=on  LabelV=Vabc_MAN7  Vpu=on  VpuLL=off  CurrentMeasurement=no  SetLabelI=on  LabelI=Iabc_MAN7  Ipu=on  Pbase=100e6  Vbase=735e3  OutputType=Magnitude  PhasorSimulation=off  PSBequivalent=0
  MIC-LTD 409 km : spsDistributedParametersLineLib/Distributed Parameters Line  Phases=3  Length=409  Frequency=60  Resistance="[0.01273  0.3864]"  Inductance="[0.9337e-3  4.1264e-3]"  Capacitance=[12.74e-9 7.751e-9]  x1=[-0.002325 7.12559654183453e-09 0 0;-0.00225 7.07279884930805e-09 0 0;-0.002175 7.01434726959888e-09 0 0;-0.0021 6.95028852800551e-09 0 0;-0.002025 6.88067383210583e-09 0 0;-0.00195 6.80555883082261e-09 0 0;-0.001875 6.72500356993856e-09 0 0;-0.0018 6.63907244409672e-09 0 0;-0.001725 6.54783414532428e-09 0 0;-0.00165 6.45136160812128e-09 0 0;-0.001575 6.3497319511579e-09 0 0;-0.0015 6.24302641562692e-09 0 0;-0.001425 6.1313303003008e-09 145223.563249357 -624254.194066257;-0.00135 6.01473289334511e-09 162813.550735245 -619899.168329279;-0.001275 5.89332740094298e-09 180273.387559806 -615048.604681913;-0.0012 5.76721087278747e-09 197589.116596627 -609706.380590524;-0.001125 5.63648412450155e-09 214746.895916856 -603876.766547311;-0.00105 5.50125165704759e-09 231733.009854226 -597564.422656545;-0.000975 5.36162157319096e-09 248533.879969153 -590774.39490935;-0.0009 5.21770549108429e-09 265136.075903129 -583512.111150015;-0.000825 5.06961845504161e-09 281526.326114745 -575783.376737061;-0.00075 4.91747884357374e-09 297691.528488763 -567594.369902525;-0.000675 4.76140827475826e-09 313618.76080974 -558951.636813174;-0.0006 4.60153150901993e-09 329295.291091853 -549862.086337602;-0.000525 4.43797634939908e-09 344708.587756655 -540332.984523383;-0.00045 4.27087353938784e-09 359846.329650622 -530371.948788708;-0.000375 4.10035665841577e-09 374696.4158945 -519986.941833135;-0.0003 3.92656201506852e-09 389246.975556559 -509186.265272327;-0.000225 3.74962853812484e-09 403486.377142037 -497978.553001871;-0.00015 3.56969766549902e-09 417403.237891176 -486372.764295473;-7.5e-05 3.38691323117761e-09 430986.432878428 -474378.17664305]  x2=[-0.002325 2.0129117581244e-08 0 0;-0.00225 2.01654662501237e-08 0 0;-0.002175 2.01856949538252e-08 0 0;-0.0021 2.0189787521832e-08 0 0;-0.002025 2.0177740682608e-08 0 0;-0.00195 2.0149564066212e-08 0 0;-0.001875 2.01052801966003e-08 0 0;-0.0018 2.00449244736204e-08 0 0;-0.001725 1.9968545144714e-08 0 0;-0.00165 1.98762032663479e-08 0 0;-0.001575 1.97679726552067e-08 0 0;-0.0015 1.96439398291852e-08 0 0;-0.001425 1.95042039382265e-08 -192622.277099833 -631827.111409279;-0.00135 1.93488766850639e-08 -174683.174298938 -637020.120753555;-0.001275 1.91780822359271e-08 -156604.43244125 -641703.905960035;-0.0012 1.89919571212853e-08 -138400.503396396 -645874.72288249;-0.001125 1.87906501267075e-08 -120085.939106726 -649529.237433687;-0.00105 1.85743221739249e-08 -101675.379954711 -652664.52825061;-0.000975 1.83431461921932e-08 -83183.5430596452 -655278.089029752;-0.0009 1.8097306980055e-08 -64625.2105130086 -657367.830530614;-0.000825 1.7837001057615e-08 -46015.2175618868 -658932.082245816;-0.00075 1.75624365094449e-08 -27368.4407499025 -659969.593736469;-0.000675 1.72738328182434e-08 -8699.7860251338 -660479.535631762;-0.0006 1.69714206893854e-08 9975.82317547212 -660461.500291947;-0.000525 1.66554418664999e-08 28643.4578556668 -659915.502134199;-0.00045 1.6326148938223e-08 47288.1953939113 -658841.97762109;-0.000375 1.59838051362834e-08 65895.1314722915 -657241.784911691;-0.0003 1.56286841250783e-08 84449.3919908021 -655116.203175571;-0.000225 1.52610697829104e-08 102936.144957474 -652466.931570246;-0.00015 1.48812559750603e-08 121340.612344843 -649296.087882902;-7.5e-05 1.44895463188746e-08 139648.081903277 -645606.206837468]  x3=[-0.002325 8.19099256173943e-12 0 0;-0.00225 8.83993320923674e-12 0 0;-0.002175 9.4818073493821e-12 0 0;-0.0021 1.01161018778089e-11 0 0;-0.002025 1.07423097491761e-11 0 0;-0.00195 1.13599303824926e-11 0 0;-0.001875 1.19684700612742e-11 0 0;-0.0018 1.25674423282125e-11 0 0;-0.001725 1.3156368374042e-11 0 0;-0.00165 1.37347774202924e-11 0 0;-0.001575 1.43022070956222e-11 0 0;-0.0015 1.48582038054309e-11 0 0;-0.001425 1.54023230944556e-11 -230.757724949157 15.8712450239567;-0.00135 1.59341300020621e-11 -231.114329922444 9.34106728403461;-0.001275 1.64531994099453e-11 -231.286185636558 2.80342243784879;-0.0012 1.69591163819626e-11 -231.273154712672 -3.73646342134005;-0.001125 1.74514764958273e-11 -231.075247567507 -10.2733624088397;-0.00105 1.79298861663978e-11 -230.692622405006 -16.8020490276174;-0.000975 1.83939629603033e-11 -230.12558508987 -23.3173043454824;-0.0009 1.88433359016555e-11 -229.374588903053 -29.8139201670203;-0.000825 1.92776457686005e-11 -228.440234179416 -36.286703196945;-0.00075 1.96965453804761e-11 -227.323267827828 -42.7304791915393;-0.000675 2.00996998753417e-11 -226.024582734101 -49.1400970948661;-0.0006 2.04867869776627e-11 -224.545217047229 -55.5104331564439;-0.000525 2.08574972559321e-11 -222.886353349506 -61.8363950270946;-0.00045 2.12115343700255e-11 -221.049317711192 -68.1129258296892;-0.000375 2.15486153080909e-11 -219.035578630467 -74.3350082015383;-0.0003 2.18684706127838e-11 -216.846745859541 -80.4976683051948;-0.000225 2.21708445966677e-11 -214.484569117842 -86.5959798044638;-0.00015 2.24554955466064e-11 -211.950936693314 -92.62506780244;-7.5e-05 2.27221959169857e-11 -209.247873932951 -98.580112738426]  x4=[-0.002325 2.37215539489519e-11 0 0;-0.00225 2.34989553984204e-11 0 0;-0.002175 2.32575721424895e-11 0 0;-0.0021 2.29975971392408e-11 0 0;-0.002025 2.27192382087139e-11 0 0;-0.00195 2.2422717866779e-11 0 0;-0.001875 2.21082731472604e-11 0 0;-0.0018 2.17761554124559e-11 0 0;-0.001725 2.1426630152201e-11 0 0;-0.00165 2.10599767716409e-11 0 0;-0.001575 2.0676488367878e-11 0 0;-0.0015 2.02764714956746e-11 0 0;-0.001425 1.98602459223981e-11 -1193.29181621004 -4540.40590051508;-0.00135 1.94281443724031e-11 -1064.45477492564 -4572.32612353389;-0.001275 1.89805122610574e-11 -934.766824780871 -4600.59129900848;-0.0012 1.85177074186218e-11 -804.331636338781 -4625.17883219004;-0.001125 1.80400998042062e-11 -673.253477493288 -4646.06906818077;-0.00105 1.75480712100299e-11 -541.63713011901 -4663.24530764563;-0.000975 1.70420149562227e-11 -409.587806310242 -4676.6938201616;-0.0009 1.65223355764112e-11 -277.211064276012 -4686.40385519356;-0.000825 1.59894484943401e-11 -144.612723958473 -4692.36765068805;-0.00075 1.54437796917893e-11 -11.8987824420492 -4694.58043927822;-0.000675 1.48857653680507e-11 120.824670779002 -4693.04045209472;-0.0006 1.43158515912367e-11 253.45153860691 -4687.74892017974;-0.000525 1.37344939417006e-11 385.875801152795 -4678.71007350293;-0.00045 1.31421571478523e-11 517.991600487337 -4665.93113758003;-0.000375 1.25393147146617e-11 649.693325261986 -4649.42232769688;-0.0003 1.19264485451462e-11 780.875695133062 -4629.19684074353;-0.000225 1.13040485551444e-11 911.433844921247 -4605.27084466477;-0.00015 1.06726122816855e-11 1041.26340843921 -4577.66346553579;-7.5e-05 1.0032644485265e-11 1170.26060192033 -4546.39677227306]  x5=0.00231306500901259  V1=ones(3,3)  V2=ones(3,3)  I1=ones(3,3)  I2=ones(3,3)  nHarmo=1  Measurements=None  Decoupling=off  VsMag0=[ 1 1 1]  VrMag0=[ 1 1 1]  VsAngle0=[0 -120 120]  VrAngle0=[0 -120 120]  IsMag0=[ 1 1 1]  IrMag0=[ 1 1 1]  IsAngle0=[0 -120 120]  IrAngle0=[0 -120 120]
      settings: AttributesFormatString=\n  LibrarySourceBlock=sps_lib/Power Grid Elements/Distributed Parameters Line
  MIC-MAN 60 km : spsDistributedParametersLineLib/Distributed Parameters Line  Phases=3  Length=60  Frequency=60  Resistance="[0.01273  0.3864]"  Inductance="[0.9337e-3  4.1264e-3]"  Capacitance=[12.74e-9 7.751e-9]  x1=[-0.000375 4.30140229284727e-09 334292.879204072 -555156.276734739;-0.0003 4.09343114002513e-09 349853.8455057 -545483.769756842;-0.000225 3.88218776098125e-09 365135.143996173 -535375.211399583;-0.00015 3.66784102044071e-09 380124.559039291 -524838.682289847;-7.5e-05 3.45056226390827e-09 394810.108326014 -513882.60516779]  x2=[-0.000375 9.59315739156434e-11 348782.647501518 -529245.722255885;-0.0003 -5.74692658953743e-11 363605.315689394 -519173.936888575;-0.000225 -2.10824165654545e-10 378137.323351256 -508687.131819744;-0.00015 -3.64010535801408e-10 392367.053822526 -497793.690040911;-7.5e-05 -5.16905921495501e-10 406283.132074387 -486502.319602757]  x3=[-0.000375 -2.33166517059242e-11 2401.79476190206 -2735.13228390528;-0.0003 -2.45578121605084e-11 2478.15848728111 -2666.13912589988;-0.000225 -2.57793414757987e-11 2552.54121068253 -2595.01469707052;-0.00015 -2.69802631799504e-11 2624.88347169532 -2521.81585319739;-7.5e-05 -2.81596172745279e-11 2695.1274410229 -2446.60110831628]  x4=[-0.000375 2.86005057799761e-11 -40.0475234765488 -1360.36447471819;-0.0003 2.94410433841714e-11 -1.57321375593878 -1360.95300908502;-0.000225 3.02580462687484e-11 36.9023535676768 -1360.45361843967;-0.00015 3.10508613341018e-11 75.3484217144753 -1358.86670198738;-7.5e-05 3.18188548159988e-11 113.734257485825 -1356.19352828487]  x5=0.000339324940197445  V1=ones(3,3)  V2=ones(3,3)  I1=ones(3,3)  I2=ones(3,3)  nHarmo=1  Measurements=None  Decoupling=off  VsMag0=[ 1 1 1]  VrMag0=[ 1 1 1]  VsAngle0=[0 -120 120]  VrAngle0=[0 -120 120]  IsMag0=[ 1 1 1]  IrMag0=[ 1 1 1]  IsAngle0=[0 -120 120]  IrAngle0=[0 -120 120]
      settings: AttributesFormatString=\n  LibrarySourceBlock=sps_lib/Power Grid Elements/Distributed Parameters Line
  Regulateurs6 : Subsystem
  Regulateurs7 : Subsystem
  "MIC7a " : PMIOPort  Side=Left
  MIC7b : PMIOPort  Port=2  Side=Left
  MIC7c : PMIOPort  Port=3  Side=Left
  QUE7a : PMIOPort  Port=4  Side=Left
  QUE7b : PMIOPort  Port=5  Side=Left
  QUE7c : PMIOPort  Port=6  Side=Left
  wires:
  Regulateurs6/1(Pm) -> "B_6 CHU-5600 MVA "/1
  Regulateurs6/2(Vf) -> "B_6 CHU-5600 MVA "/2
  "B_6 CHU-5600 MVA "/1 -> Regulateurs6/1(m)
  Regulateurs7/1(Pm) -> B_7 MAN 5000 MVA/1
  Regulateurs7/2(Vf) -> B_7 MAN 5000 MVA/2
  B_7 MAN 5000 MVA/1 -> Regulateurs7/1(m)
  connections:
  "Cs PER "/RConn3 -- MIC-LTD 409 km/LConn3
  "Cs PER "/RConn2 -- MIC-LTD 409 km/LConn2
  "Cs PER "/RConn1 -- MIC-LTD 409 km/LConn1
  Cs BER/RConn3 -- MAN-LEV 3*379km/LConn3
  Cs BER/RConn2 -- MAN-LEV 3*379km/LConn2
  Cs BER/RConn1 -- MAN-LEV 3*379km/LConn1
  Cs ARNS2/RConn3 -- ARN-MAN 2*169km/LConn3
  Cs ARNS2/RConn2 -- ARN-MAN 2*169km/LConn2
  Cs ARNS2/RConn1 -- ARN-MAN 2*169km/LConn1
  CHU-ARN 3*450km/RConn3 -- "Cs MTG+ARNN "/LConn3
  CHU-ARN 3*450km/RConn2 -- "Cs MTG+ARNN "/LConn2
  CHU-ARN 3*450km/RConn1 -- "Cs MTG+ARNN "/LConn1
  Load Flow Bus2/LConn1 -- 5600 MVA 13.8 kV/735 kV1/RConn3 -- CHU-ARN 3*450km/LConn3 -- CHU 330 Mvar/LConn3
  5600 MVA 13.8 kV/735 kV1/RConn2 -- CHU-ARN 3*450km/LConn2 -- CHU 330 Mvar/LConn2
  5600 MVA 13.8 kV/735 kV1/RConn1 -- CHU-ARN 3*450km/LConn1 -- CHU 330 Mvar/LConn1
  "B_6 CHU-5600 MVA "/RConn3 -- Load Flow Bus1/LConn1 -- 5600 MVA 13.8 kV/735 kV1/LConn3 -- 280 MW/LConn3
  5600 MVA 13.8 kV/735 kV1/LConn2 -- "B_6 CHU-5600 MVA "/RConn2 -- 280 MW/LConn2
  5600 MVA 13.8 kV/735 kV1/LConn1 -- "B_6 CHU-5600 MVA "/RConn1 -- 280 MW/LConn1
  "Cs ARNS1 "/RConn1 -- ARN-MIC 180km/LConn1
  "Cs ARNS1 "/RConn2 -- ARN-MIC 180km/LConn2
  "Cs ARNS1 "/RConn3 -- ARN-MIC 180km/LConn3
  "Cs PER "/LConn3 -- Load Flow Bus6/LConn1 -- MIC7c/RConn1 -- MIC-MAN 60 km/LConn3 -- ARN-MIC 180km/RConn3
  "Cs PER "/LConn2 -- MIC7b/RConn1 -- ARN-MIC 180km/RConn2 -- MIC-MAN 60 km/LConn2
  "Cs PER "/LConn1 -- "MIC7a "/RConn1 -- ARN-MIC 180km/RConn1 -- MIC-MAN 60 km/LConn1
  ARN-MAN 2*169km/RConn1 -- MAN7/LConn1
  ARN-MAN 2*169km/RConn2 -- MAN7/LConn2
  ARN-MAN 2*169km/RConn3 -- MAN7/LConn3
  Cs BER/LConn1 -- 5000 MVA 13.8 kV/735 kV2/RConn1 -- MIC-MAN 60 km/RConn1 -- MAN-MIC 1650 Mvar/LConn1 -- MAN7/RConn1
  Cs BER/LConn2 -- 5000 MVA 13.8 kV/735 kV2/RConn2 -- MIC-MAN 60 km/RConn2 -- MAN-MIC 1650 Mvar/LConn2 -- MAN7/RConn2
  Cs BER/LConn3 -- Load Flow Bus5/LConn1 -- 5000 MVA 13.8 kV/735 kV2/RConn3 -- MIC-MAN 60 km/RConn3 -- MAN-MIC 1650 Mvar/LConn3 -- MAN7/RConn3
  B_7 MAN 5000 MVA/RConn1 -- 5000 MVA 13.8 kV/735 kV2/LConn1 -- 250 MW/LConn1
  B_7 MAN 5000 MVA/RConn2 -- 5000 MVA 13.8 kV/735 kV2/LConn2 -- 250 MW/LConn2
  B_7 MAN 5000 MVA/RConn3 -- 5000 MVA 13.8 kV/735 kV2/LConn3 -- Load Flow Bus3/LConn1 -- 250 MW/LConn3
  MIC-LTD 409 km/RConn2 -- MAN-LEV 3*379km/RConn2 -- QUE7b/RConn1
  Cs ARNS2/LConn1 -- ARN 990 Mvar/LConn1 -- "Cs MTG+ARNN "/RConn1 -- "Cs ARNS1 "/LConn1
  Cs ARNS2/LConn2 -- ARN 990 Mvar/LConn2 -- "Cs MTG+ARNN "/RConn2 -- "Cs ARNS1 "/LConn2
  Cs ARNS2/LConn3 -- Load Flow Bus4/LConn1 -- "Cs ARNS1 "/LConn3 -- ARN 990 Mvar/LConn3 -- "Cs MTG+ARNN "/RConn3
  MIC-LTD 409 km/RConn1 -- QUE7a/RConn1 -- MAN-LEV 3*379km/RConn1
  MIC-LTD 409 km/RConn3 -- QUE7c/RConn1 -- MAN-LEV 3*379km/RConn3
